simulink model "IM_Updated"  (R2022b)
settings: Solver=FixedStepAuto  StartTime=0.0  StopTime=2  FixedStep=0.0001  RelTol=1e-3
values from neighbouring files (symbols this model uses):
  f = 6.32E-4    (= 0.000632)    [init.m]    (also in kttestm.m)
  fs = 50    [init.m]    (also in kttestm.m)
  J = 4.5E-2    (= 0.045)    [init.m]    (also in kttestm.m)
  Lr = 0.2395    [init.m]    (also in kttestm.m)
  Ls = 0.256    [init.m]    (also in kttestm.m)
  Msr = 0.236    [init.m]    (also in kttestm.m)
  P = 2    [init.m]    (also in kttestm.m)
  Rr = 1.09    [init.m]    (also in kttestm.m)
  Rs = 3.36    [init.m]    (also in kttestm.m)
  vit_rad_s = temp(ind)    [init.m]
  Vmax = 220*sqrt(2)    [init.m]    (also in kttestm.m)
settings Model: SimulationMode=accelerator  Creator=guillaume  LastModifiedBy=ZinouAb
settings SolverCC: AlgebraicLoopSolver=TrustRegion
settings DataIOCC: ReturnWorkspaceOutputs=off
settings DebuggingCC: UnconnectedInputMsg=warning  UnconnectedOutputMsg=warning  UnconnectedLineMsg=warning  SFMachineParentedDataDiag=warning  ArithmeticOperatorsInVariantConditions=warning
settings ModelReferenceCC: EnableRefExpFcnMdlSchedulingChecks=on
settings SFSimCC: SimUseLocalCustomCode=off  CustomCodeUndefinedFunction=UseInterfaceOnly
settings RTWCC: RTWUseLocalCustomCode=off  DLArmComputeVersion=19.05
settings CodeAppCC: StateflowObjectComments=on

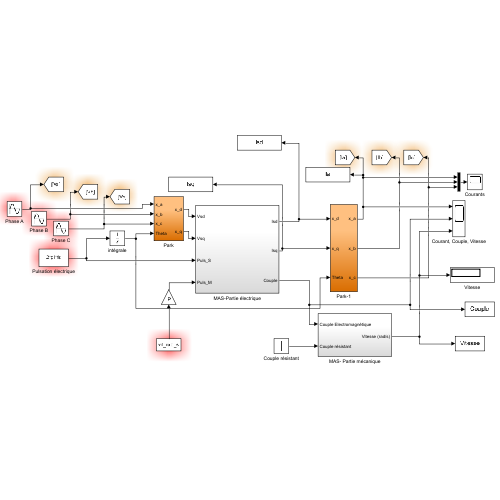
[thumbnail: Simulink's stored preview of the top-level diagram]
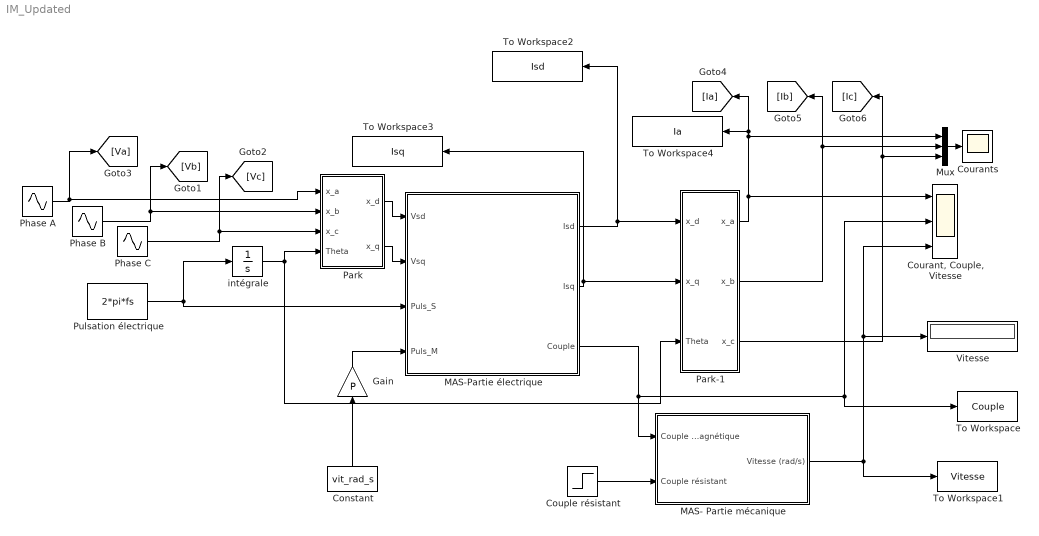
== system IM_Updated ==
  Constant : Constant  Value=vit_rad_s
  Couple résistant : Step  After=20  SampleTime=0
  "Courant, Couple, Vitesse" : Scope  NumInputPorts=3
  Courants : Scope
  Gain : Gain  Gain=P
  MAS- Partie mécanique : Subsystem
  MAS-Partie électrique : Subsystem
  Mux : Mux  Inputs=3
  Park : Subsystem
  Park-1 : Subsystem
  Phase A : Sin  Amplitude=Vmax  Frequency=2*pi*fs  SampleTime=0
  Phase B : Sin  Amplitude=Vmax  Frequency=2*pi*fs  Phase=-2*pi/3  SampleTime=0
  Phase C : Sin  Amplitude=Vmax  Frequency=2*pi*fs  Phase=2*pi/3  SampleTime=0
  Pulsation électrique : Constant  Value=2*pi*fs
  To Workspace : ToWorkspace  VariableName=Couple  SampleTime=-1
      settings: Save2DSignal=2-D array (concatenate along first dimension)
  To Workspace1 : ToWorkspace  VariableName=Vitesse  SampleTime=-1
      settings: Save2DSignal=2-D array (concatenate along first dimension)
  To Workspace2 : ToWorkspace  VariableName=Isd  SaveFormat=Timeseries  SampleTime=-1
  To Workspace3 : ToWorkspace  VariableName=Isq  SaveFormat=Timeseries  SampleTime=-1
  To Workspace4 : ToWorkspace  VariableName=Ia  SaveFormat=Timeseries  SampleTime=-1
  Vitesse : Display
  intégrale : Integrator
  wires:
  Couple résistant/1 -> MAS- Partie mécanique/2(Couple résistant)
  Pulsation électrique/1 -> intégrale/1, MAS-Partie électrique/3(Puls_S)
  Phase C/1 -> [Vc], Park/3(x_c)
  Phase B/1 -> [Vb], Park/2(x_b)
  Park/1(x_d) -> MAS-Partie électrique/1(Vsd)
  Gain/1 -> MAS-Partie électrique/4(Puls_M)
  Park/2(x_q) -> MAS-Partie électrique/2(Vsq)
  MAS-Partie électrique/1(Isd) -> To Workspace2/1, Park-1/1(x_d)
  MAS-Partie électrique/2(Isq) -> To Workspace3/1, Park-1/2(x_q)
  Park-1/1(x_a) -> "Courant, Couple, Vitesse"/1, To Workspace4/1, [Ia], Mux/1
  Park-1/3(x_c) -> Mux/3, [Ic]
  Park-1/2(x_b) -> Mux/2, [Ib]
  Mux/1 -> Courants/1
  MAS-Partie électrique/3(Couple) -> MAS- Partie mécanique/1(Couple Electromagnétique), "Courant, Couple, Vitesse"/2, To Workspace/1
  MAS- Partie mécanique/1(Vitesse (rad/s)) -> Vitesse/1, "Courant, Couple, Vitesse"/3, To Workspace1/1
  intégrale/1 -> Park-1/3(Theta), Park/4(Theta)
  Phase A/1 -> [Va], Park/1(x_a)
  Constant/1 -> Gain/1

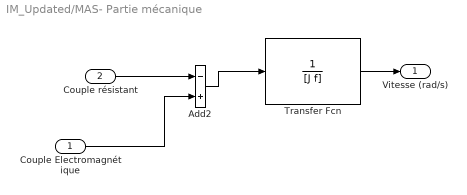
== system IM_Updated/MAS- Partie mécanique ==
  Couple Electromagnétique : Inport
  Couple résistant : Inport  Port=2
  Add2 : Sum  Inputs=-+
  Transfer Fcn : TransferFcn  Denominator=[J f]
  Vitesse (rad/s) : Outport
  wires:
  Couple Electromagnétique/1 -> Add2/2
  Couple résistant/1 -> Add2/1
  Add2/1 -> Transfer Fcn/1
  Transfer Fcn/1 -> Vitesse (rad/s)/1

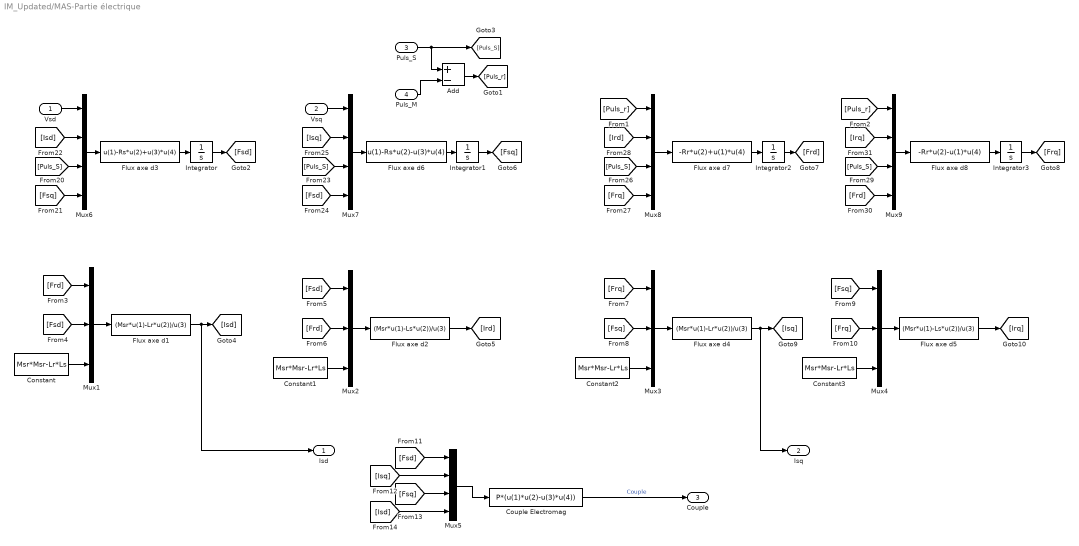
== system IM_Updated/MAS-Partie électrique ==
  Vsd : Inport
  Vsq : Inport  Port=2
  Puls_S : Inport  Port=3
  Puls_M : Inport  Port=4
  Add : Sum  Inputs=+-
  Constant{,1..3} (4 alike) : Constant  Value=Msr*Msr-Lr*Ls
  Couple Electromag : Fcn  Expr=P*(u(1)*u(2)-u(3)*u(4))
  Flux axe d1 : Fcn  Expr=(Msr*u(1)-Lr*u(2))/u(3)
  Flux axe d2 : Fcn  Expr=(Msr*u(1)-Ls*u(2))/u(3)
  Flux axe d3 : Fcn  Expr=u(1)-Rs*u(2)+u(3)*u(4)
  Flux axe d4 : Fcn  Expr=(Msr*u(1)-Lr*u(2))/u(3)
  Flux axe d5 : Fcn  Expr=(Msr*u(1)-Ls*u(2))/u(3)
  Flux axe d6 : Fcn  Expr=u(1)-Rs*u(2)-u(3)*u(4)
  Flux axe d7 : Fcn  Expr=-Rr*u(2)+u(1)*u(4)
  Flux axe d8 : Fcn  Expr=-Rr*u(2)-u(1)*u(4)
  Integrator{,1..3} (4 alike) : Integrator
  Mux{1..4} (4 alike) : Mux  Inputs=3
  Mux{5..9} (5 alike) : Mux
  Isd : Outport
  Isq : Outport  Port=2
  Couple : Outport  Port=3
  wires:
  Puls_S/1 -> Add/1, [Puls_S]
  Mux6/1 -> Flux axe d3/1
  Vsd/1 -> Mux6/1
  [Isd] -> Mux6/2
  [Puls_S] -> Mux6/3
  [Fsq] -> Mux6/4
  Flux axe d3/1 -> Integrator/1
  Integrator/1 -> [Fsd]
  Mux7/1 -> Flux axe d6/1
  Vsq/1 -> Mux7/1
  [Isq] -> Mux7/2
  [Puls_S] -> Mux7/3
  [Fsd] -> Mux7/4
  Flux axe d6/1 -> Integrator1/1
  Integrator1/1 -> [Fsq]
  Mux8/1 -> Flux axe d7/1
  [Ird] -> Mux8/2
  [Puls_S] -> Mux8/3
  [Frq] -> Mux8/4
  Flux axe d7/1 -> Integrator2/1
  Integrator2/1 -> [Frd]
  Mux9/1 -> Flux axe d8/1
  [Puls_r] -> Mux8/1
  [Irq] -> Mux9/2
  [Puls_S] -> Mux9/3
  [Frd] -> Mux9/4
  Flux axe d8/1 -> Integrator3/1
  Integrator3/1 -> [Frq]
  [Puls_r] -> Mux9/1
  [Frd] -> Mux1/1
  [Fsd] -> Mux1/2
  Mux1/1 -> Flux axe d1/1
  Constant/1 -> Mux1/3
  Flux axe d1/1 -> Isd/1, [Isd]
  [Fsd] -> Mux2/1
  [Frd] -> Mux2/2
  Mux2/1 -> Flux axe d2/1
  Constant1/1 -> Mux2/3
  Flux axe d2/1 -> [Ird]
  [Frq] -> Mux3/1
  [Fsq] -> Mux3/2
  Mux3/1 -> Flux axe d4/1
  Constant2/1 -> Mux3/3
  Flux axe d4/1 -> Isq/1, [Isq]
  [Fsq] -> Mux4/1
  [Frq] -> Mux4/2
  Mux4/1 -> Flux axe d5/1
  Constant3/1 -> Mux4/3
  Flux axe d5/1 -> [Irq]
  Mux5/1 -> Couple Electromag/1
  Couple Electromag/1 -> Couple/1  "Couple"
  [Isd] -> Mux5/4
  [Fsd] -> Mux5/1
  [Isq] -> Mux5/2
  [Fsq] -> Mux5/3
  Puls_M/1 -> Add/2
  Add/1 -> [Puls_r]

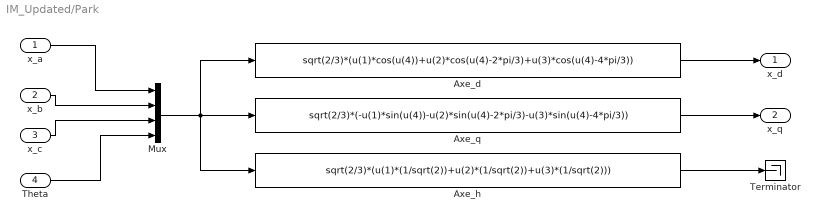
== system IM_Updated/Park ==
  x_a : Inport
  x_b : Inport  Port=2
  x_c : Inport  Port=3
  Theta : Inport  Port=4
  " Axe_h" : Fcn  Expr=sqrt(2/3)*(u(1)*(1/sqrt(2))+u(2)*(1/sqrt(2))+u(3)*(1/sqrt(2)))
  " Axe_q" : Fcn  Expr=sqrt(2/3)*(-u(1)*sin(u(4))-u(2)*sin(u(4)-2*pi/3)-u(3)*sin(u(4)-4*pi/3))
  Axe_d : Fcn  Expr=sqrt(2/3)*(u(1)*cos(u(4))+u(2)*cos(u(4)-2*pi/3)+u(3)*cos(u(4)-4*pi/3))
  Mux : Mux
  Terminator : Terminator
  x_d : Outport
  x_q : Outport  Port=2
  wires:
  x_a/1 -> Mux/1
  x_b/1 -> Mux/2
  x_c/1 -> Mux/3
  Theta/1 -> Mux/4
  Mux/1 -> " Axe_q"/1, " Axe_h"/1, Axe_d/1
  " Axe_h"/1 -> Terminator/1
  " Axe_q"/1 -> x_q/1
  Axe_d/1 -> x_d/1

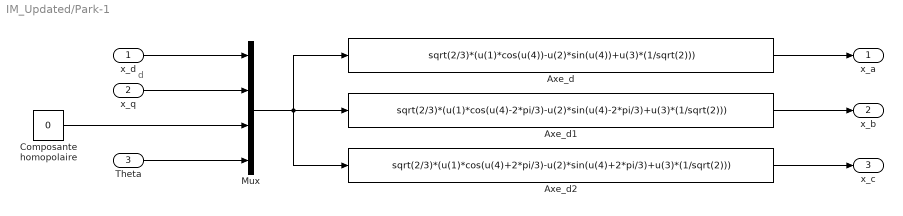
== system IM_Updated/Park-1 ==
  note: d
  x_d : Inport
  x_q : Inport  Port=2
  Theta : Inport  Port=3
  Axe_d : Fcn  Expr=sqrt(2/3)*(u(1)*cos(u(4))-u(2)*sin(u(4))+u(3)*(1/sqrt(2)))
  Axe_d1 : Fcn  Expr=sqrt(2/3)*(u(1)*cos(u(4)-2*pi/3)-u(2)*sin(u(4)-2*pi/3)+u(3)*(1/sqrt(2)))
  Axe_d2 : Fcn  Expr=sqrt(2/3)*(u(1)*cos(u(4)+2*pi/3)-u(2)*sin(u(4)+2*pi/3)+u(3)*(1/sqrt(2)))
  Composante homopolaire : Constant  Value=0
  Mux : Mux
  x_a : Outport
  x_b : Outport  Port=2
  x_c : Outport  Port=3
  wires:
  x_d/1 -> Mux/1
  x_q/1 -> Mux/2
  Mux/1 -> Axe_d1/1, Axe_d2/1, Axe_d/1
  Axe_d2/1 -> x_c/1
  Axe_d1/1 -> x_b/1
  Axe_d/1 -> x_a/1
  Theta/1 -> Mux/4
  Composante homopolaire/1 -> Mux/3
